simulink model "MotorBench"  (R2024b)
settings: Solver=VariableStepAuto  StartTime=0.0  StopTime=50.0  RelTol=1e-3
model workspace (MATLAB code in the model file):
  | AllParams;
settings Model: Creator=Marij  LastModifiedBy=marijn
settings OptimizationCC: UseDivisionForNetSlopeComputation=on

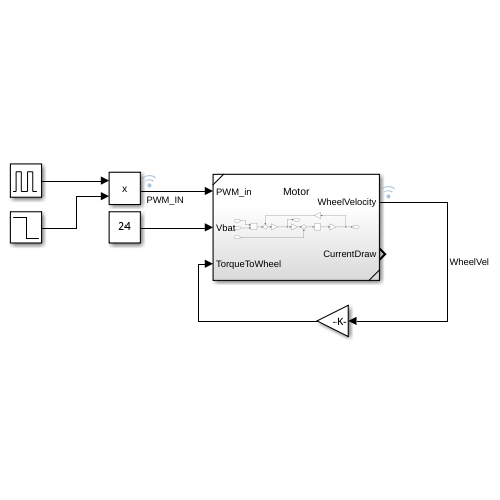
[thumbnail: Simulink's stored preview of the top-level diagram]
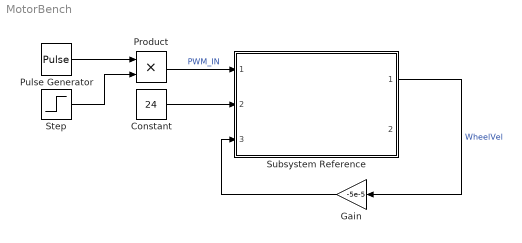
== system MotorBench ==
  Constant : Constant  Value=24
  Gain : Gain  Gain=-5e-5
  Product : Product
  Pulse Generator : DiscretePulseGenerator  PulseType=Time based  Period=10  PulseWidth=50  PhaseDelay=2.5
  Step : Step  Time=10  Before=1  After=0  SampleTime=0
  Subsystem Reference : Subsystem  ReferencedSubsystem=Motor
  wires:
  Subsystem Reference/1 -> Gain/1  "WheelVel"
  Gain/1 -> Subsystem Reference/3
  Constant/1 -> Subsystem Reference/2
  Step/1 -> Product/2
  Pulse Generator/1 -> Product/1
  Product/1 -> Subsystem Reference/1  "PWM_IN"
